simulink model "parameters_identification_21_a"  (R2024a)
settings: Solver=ode4  StartTime=0.0  StopTime=5  RelTol=1e-3
values from neighbouring files (symbols this model uses):
  f = (1-phi_m)/gamma_m    [electrical_mechanical_parameters.m]
  ia = V(:,3)    [electrical_mechanical_parameters.m]
  J = -(f*h)/log(phi_m)    [electrical_mechanical_parameters.m]
  Ka = Kg    [electrical_mechanical_parameters.m]
  La = -(Ra*h)/(log(phi_e))    [electrical_mechanical_parameters.m]
  Ra = (1-phi_e)/gamma_e    [electrical_mechanical_parameters.m]
  vt = V(:,2)    [electrical_mechanical_parameters.m]
undefined symbols (not defined in the file or in its folder): Kg, Kt
settings Model: Creator=Guilherme  LastModifiedBy=Guilherme

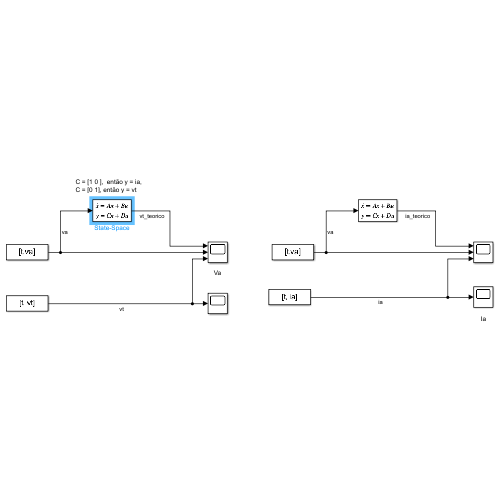
[thumbnail: Simulink's stored preview of the top-level diagram]
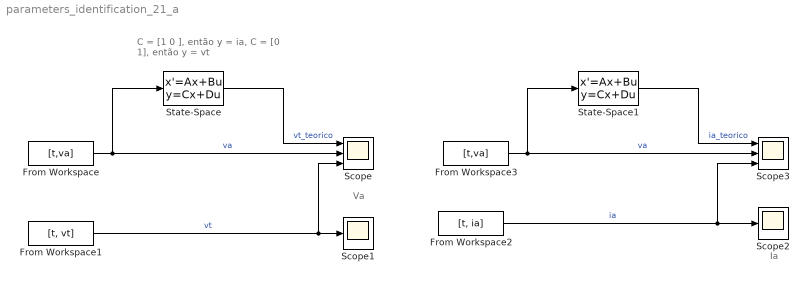
== system parameters_identification_21_a ==
  note: Ia
  note: Va
  note: C = [1 0 ],  então y = ia,
      | C = [0 1], então y = vt
  From Workspace : FromWorkspace  VariableName=[t,va]
  From Workspace1 : FromWorkspace  VariableName=[t, vt]
  From Workspace2 : FromWorkspace  VariableName=[t, ia]
  From Workspace3 : FromWorkspace  VariableName=[t,va]
  Scope : Scope  NumInputPorts=3
  Scope1 : Scope
  Scope2 : Scope
  Scope3 : Scope  NumInputPorts=3
  State-Space : StateSpace  A=[-Ra/La, -Kg/(Kt*La); (Ka*Kt)/J, -f/J]  B=[1/La; 0]  C=[0, 1]  D=[0]  InitialCondition=vt(1)
  State-Space1 : StateSpace  A=[-Ra/La, -Kg/(Kt*La); (Ka*Kt)/J, -f/J]  B=[1/La; 0]  C=[1, 0]  D=[0]  InitialCondition=ia(1)
  wires:
  From Workspace/1 -> State-Space/1, Scope/2  "va"
  From Workspace1/1 -> Scope/3, Scope1/1  "vt"
  From Workspace2/1 -> Scope3/3, Scope2/1  "ia"
  State-Space/1 -> Scope/1  "vt_teorico"
  State-Space1/1 -> Scope3/1  "ia_teorico"
  From Workspace3/1 -> State-Space1/1, Scope3/2  "va"
